simulink model "es1sim"  (R2023b)
settings: Solver=VariableStepAuto  StartTime=0.0  StopTime=Tfin  RelTol=1e-3
values from neighbouring files (symbols this model uses):
  IJ = inv(J)    [es1.m]    (also in es2.m)
  J = diag([10000,9000,12000])    [es1.m]    (also in es2.m = [399 -2.81 -1.31)
  q0 = [0.6853,0.6953,0.1531,0.1531]'    [es1.m]    (also in es2.m = [0 0 1 0]')
  q_r = [1 0 0 0]'    [es1.m]
  w0 = [0.53, 0.53,0.053]'    [es1.m]    (also in es2.m = [0.1 -0.9 0.12]')
libraries: vrlib x1
settings Model: Creator=luigi  LastModifiedBy=luigi

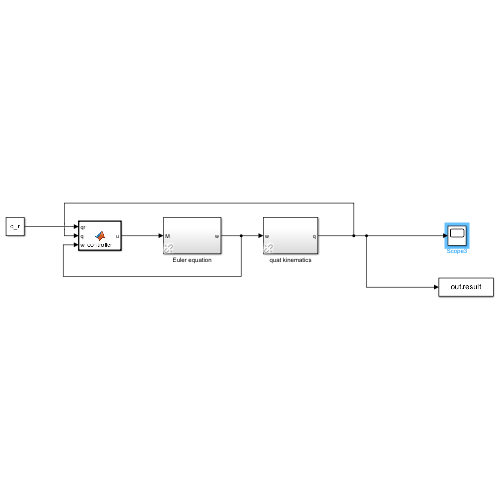
[thumbnail: Simulink's stored preview of the top-level diagram]
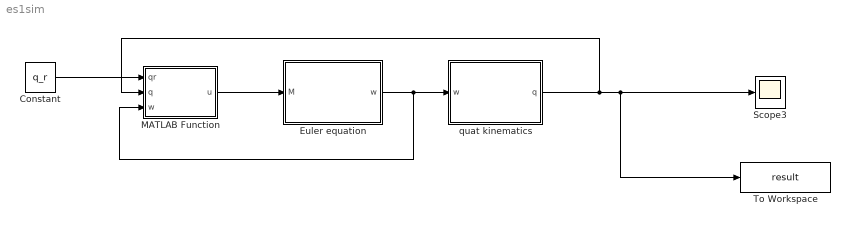
== system es1sim ==
  Constant : Constant  Value=q_r
  Euler equation : Subsystem  AncestorBlock=lib_rotations_2014/Euler equation
  MATLAB Function : MATLAB Function  TreatAsAtomicUnit=on
  Scope3 : Scope
  To Workspace : ToWorkspace  VariableName=result  SaveFormat=Timeseries  SampleTime=-1
  quat kinematics : Subsystem  AncestorBlock=lib_rotations_2014/quat kinematics
  wires:
  Euler equation/1(w) -> MATLAB Function/3(w), quat kinematics/1(w)
  quat kinematics/1(q) -> MATLAB Function/2(q), Scope3/1, To Workspace/1
  Constant/1 -> MATLAB Function/1(qr)
  MATLAB Function/1(u) -> Euler equation/1(M)

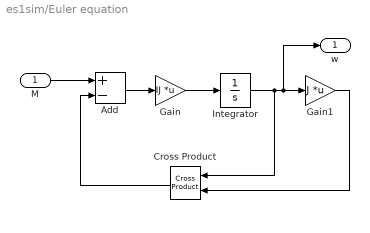
== system es1sim/Euler equation ==
  M : Inport
  Add : Sum  Inputs=+-
  Cross Product : vrlib/Utilities/Cross Product
  Gain : Gain  Gain=IJ  Multiplication=Matrix(K*u)
  Gain1 : Gain  Gain=J  Multiplication=Matrix(K*u)
  Integrator : Integrator  InitialCondition=w0
  w : Outport  PortDimensions=3  VectorParamsAs1DForOutWhenUnconnected=off
  wires:
  Cross Product/1 -> Add/2
  Add/1 -> Gain/1
  Gain1/1 -> Cross Product/2
  Gain/1 -> Integrator/1
  Integrator/1 -> Gain1/1, w/1, Cross Product/1
  M/1 -> Add/1

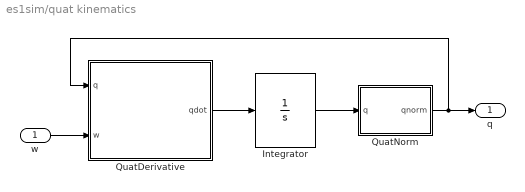
== system es1sim/quat kinematics ==
  w : Inport  PortDimensions=3
  Integrator : Integrator  InitialCondition=q0
  QuatDerivative : MATLAB Function  TreatAsAtomicUnit=on
  QuatNorm : MATLAB Function  TreatAsAtomicUnit=on
  q : Outport  PortDimensions=4  VectorParamsAs1DForOutWhenUnconnected=off
  wires:
  w/1 -> QuatDerivative/2(w)
  QuatDerivative/1(qdot) -> Integrator/1
  QuatNorm/1(qnorm) -> q/1, QuatDerivative/1(q)
  Integrator/1 -> QuatNorm/1(q)

== matlab function es1sim/quat kinematics/QuatDerivative ==
  data: q input; qdot output; w input
function qdot= QuatDerivative(q,w)
%#codegen
omegaq=[0; w];
Q=[q(1) -q(2) -q(3) -q(4);
    q(2) q(1) -q(4) q(3);
    q(3) q(4) q(1) -q(2);
    q(4) -q(3) q(2) q(1)];
qdot=Q*omegaq/2;

== matlab function es1sim/quat kinematics/QuatNorm ==
  data: q input; qnorm output
function qnorm = QuatNorm(q)
%#codegen
qnorm=zeros(4,1);
q2=sqrt(q'*q);
qnorm=q/q2;

== matlab function es1sim/MATLAB Function ==
  data: qr input; u output; q input; w input
function u = controller(qr,q,w)

qinv = [q(1); -q(2:end)];
qtilde = quatprod(qinv,qr);

kp = 500;
kd = 1000;

u = kp*qtilde(2:4) - kd*w;

end

%% Quatprod
function r = quatprod(q,p)

qq=[0 -q(4) q(3);
    q(4) 0 -q(2);
    -q(3) q(2) 0];

Q=[q(1) -q(2:4)'; 
    q(2:4) q(1)*eye(3)+qq];

r=Q*p;

end
